simulink model "LQR_controller"  (R2021b)
settings: Solver=VariableStepAuto  StartTime=0.0  StopTime=10  RelTol=1e-3
values from neighbouring files (symbols this model uses):
  A_sys = subs(A_sys,[mb mB mw rb rw l Ib IB Iw g],[4 4.906 1.415 0.12 0.05 0.208 0.01165 0.3 7.937*10^-4 -9.81])    [vanderblonk_2d.m]
  B_sys = subs(B_sys,[mb mB mw rb rw l Ib IB Iw g IB_xy Iw_xy],[4 4.9064 1.415 0.12 0.05 0.208 0.01165 0.3 7.937*10^-4 -9.81 0.3 1.176*10^-3])    [vanderblonk_2d.m]
  C_sys = eye(8)    [vanderblonk_2d.m]
  D_sys = zeros(8,3)    [vanderblonk_2d.m]
  K = lqr(double(A_sys),double(B_sys),Q,R)    [vanderblonk_2d.m]
settings Model: Creator=matas  LastModifiedBy=matas

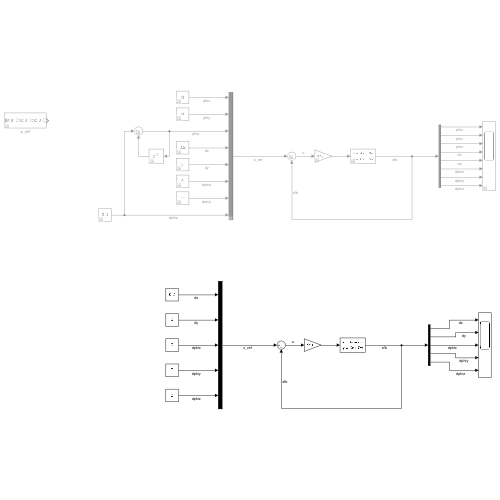
[thumbnail: Simulink's stored preview of the top-level diagram]
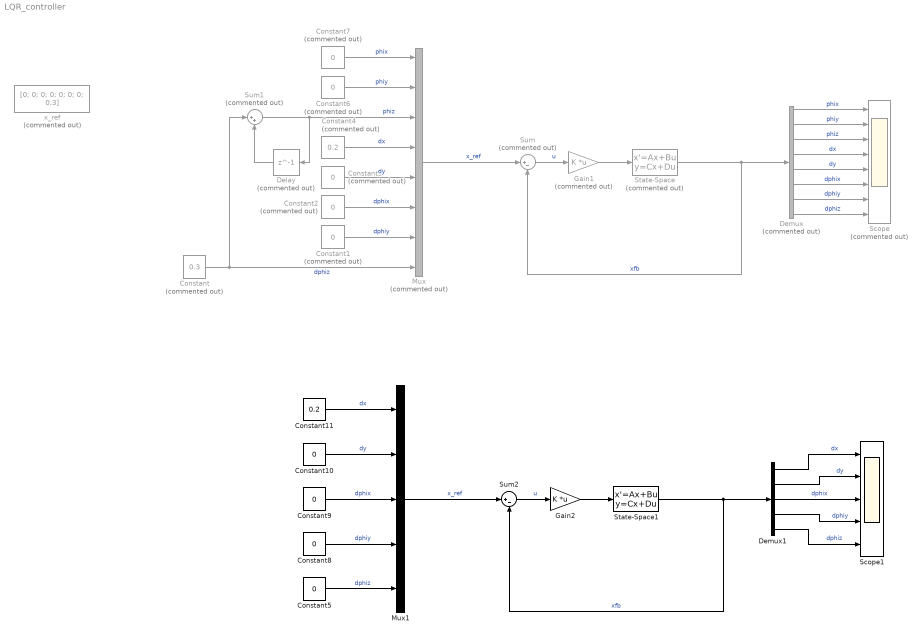
== system LQR_controller ==
  Constant : Constant  Commented=on  Value=0.3
  Constant{1..3,6..7} (5 alike) : Constant  Commented=on  Value=0
  Constant{5,8..10} (4 alike) : Constant  Value=0
  Constant11 : Constant  Value=0.2
  Constant4 : Constant  Commented=on  Value=0.2
  Delay : Delay  Commented=on  DelayLength=1  SampleTime=1
  Demux : Demux  Commented=on  Outputs=8
  Demux1 : Demux  Outputs=5
  Gain1 : Gain  Commented=on  Gain=K  Multiplication=Matrix(K*u)
  Gain2 : Gain  Gain=K  Multiplication=Matrix(K*u)
  Mux : Mux  Commented=on  Inputs=8
  Mux1 : Mux  Inputs=5
  Scope : Scope  Commented=on  NumInputPorts=8
  Scope1 : Scope  NumInputPorts=5
  State-Space : StateSpace  Commented=on  A=double(A_sys)  B=double(B_sys)  C=C_sys  D=D_sys  InitialCondition=0  AllowTunableDMatrix=on  ContinuousStateAttributes={'phix', 'phiy', 'phiz', 'dx', 'dy', 'dphix', 'dphiy', 'dphiz'}
  State-Space1 : StateSpace  A=double(A_sys)  B=double(B_sys)  C=C_sys  D=D_sys  InitialCondition=0  AllowTunableDMatrix=on  ContinuousStateAttributes={'phix', 'phiy', 'phiz', 'dx', 'dy', 'dphix', 'dphiy', 'dphiz'}
  Sum : Sum  Commented=on  Inputs=|+-
  Sum1 : Sum  Commented=on  Inputs=|++
  Sum2 : Sum  Inputs=|+-
  x_ref : Constant  Commented=on  Value=[0; 0; 0; 0; 0; 0; 0; 0.3]  VectorParams1D=off
  wires:
  State-Space/1 -> Sum/2, Demux/1  "xfb"
  Sum/1 -> Gain1/1  "u"
  Demux/1 -> Scope/1  "phix"
  Demux/2 -> Scope/2  "phiy"
  Demux/3 -> Scope/3  "phiz"
  Demux/4 -> Scope/4  "dx"
  Demux/5 -> Scope/5  "dy"
  Demux/6 -> Scope/6  "dphix"
  Demux/7 -> Scope/7  "dphiy"
  Demux/8 -> Scope/8  "dphiz"
  Gain1/1 -> State-Space/1
  Mux/1 -> Sum/1  "x_ref"
  Constant7/1 -> Mux/1  "phix"
  Constant6/1 -> Mux/2  "phiy"
  Sum1/1 -> Mux/3, Delay/1  "phiz"
  Constant4/1 -> Mux/4  "dx"
  Constant3/1 -> Mux/5  "dy"
  Constant2/1 -> Mux/6  "dphix"
  Constant1/1 -> Mux/7  "dphiy"
  Delay/1 -> Sum1/2
  Constant/1 -> Mux/8, Sum1/1  "dphiz"
  Constant9/1 -> Mux1/3  "dphix"
  Constant5/1 -> Mux1/5  "dphiz"
  Gain2/1 -> State-Space1/1
  Sum2/1 -> Gain2/1  "u"
  Constant10/1 -> Mux1/2  "dy"
  Mux1/1 -> Sum2/1  "x_ref"
  State-Space1/1 -> Demux1/1, Sum2/2  "xfb"
  Constant11/1 -> Mux1/1  "dx"
  Constant8/1 -> Mux1/4  "dphiy"
  Demux1/1 -> Scope1/1  "dx"
  Demux1/2 -> Scope1/2  "dy"
  Demux1/3 -> Scope1/3  "dphix"
  Demux1/4 -> Scope1/4  "dphiy"
  Demux1/5 -> Scope1/5  "dphiz"
